simulink subsystem "Mission_File_Parser"  (R2025b)
settings: Solver=VariableStepAuto  StartTime=0.0  StopTime=10.0  RelTol=1e-3
undefined symbols (not defined in the file or in its folder): mission_file
settings Model: Creator=koryh  LastModifiedBy=koryh

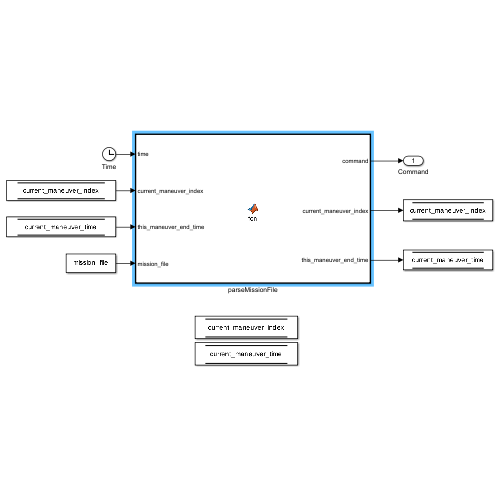
[thumbnail: Simulink's stored preview of the top-level diagram]
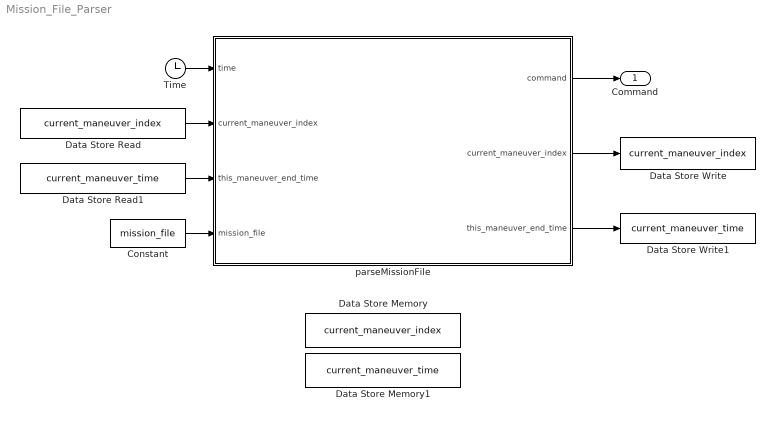
== system Mission_File_Parser ==
  Constant : Constant  Value=mission_file
  Data Store Memory : DataStoreMemory  DataStoreName=current_maneuver_index  WriteAfterWriteMsg=warning  InitialValue=1  ShowAdditionalParam=off
  Data Store Memory1 : DataStoreMemory  DataStoreName=current_maneuver_time  WriteAfterWriteMsg=warning  ShowAdditionalParam=off
  Data Store Read : DataStoreRead  DataStoreName=current_maneuver_index  IndexOptions=Index vector (dialog)  Indices=1  OutputSizes=1
  Data Store Read1 : DataStoreRead  DataStoreName=current_maneuver_time  IndexOptions=Index vector (dialog)  Indices=1  OutputSizes=1
  Data Store Write : DataStoreWrite  DataStoreName=current_maneuver_index  IndexOptions=Index vector (dialog)  Indices=1  OutputSizes=1
  Data Store Write1 : DataStoreWrite  DataStoreName=current_maneuver_time  IndexOptions=Index vector (dialog)  Indices=1  OutputSizes=1
  Time : Clock
  parseMissionFile : MATLAB Function  TreatAsAtomicUnit=on
  Command : Outport
  wires:
  Time/1 -> parseMissionFile/1(time)
  parseMissionFile/3(this_maneuver_end_time) -> Data Store Write1/1
  Constant/1 -> parseMissionFile/4(mission_file)
  Data Store Read/1 -> parseMissionFile/2("current_maneuver_index ")
  parseMissionFile/2(current_maneuver_index) -> Data Store Write/1
  Data Store Read1/1 -> parseMissionFile/3("this_maneuver_end_time ")
  parseMissionFile/1(command) -> Command/1

== matlab function Mission_File_Parser/parseMissionFile ==
  data: command output; time input; current_maneuver_index input; this_maneuver_end_time input; current_maneuver_index output; this_maneuver_end_time output; mission_file input
function [command, current_maneuver_index, this_maneuver_end_time] = ...
    fcn(time,current_maneuver_index, this_maneuver_end_time, mission_file)


[command, current_maneuver_index, this_maneuver_end_time] = ...
    parseMissionFile(mission_file,time,current_maneuver_index,...
    this_maneuver_end_time); %see utils
